simulink model "NFBLB_OSC_NON_LIN"  (R2021a)
settings: Solver=VariableStepAuto  StartTime=0.0  StopTime=85  RelTol=1e-3
model workspace (MATLAB code in the model file):
  | Kab=40;
  | Kia=0.5;
  | Kbc=20;
  | Fb=2;
  | kfb=1;
  | Kca=8;
  | Fc=0.5;
  | In=0.3;
  | x_star=[0.0069;0.5363;0.1000];
settings Model: Creator=priya  LastModifiedBy=Priyan_PC
settings SolverCC: AlgebraicLoopSolver=TrustRegion
settings DebuggingCC: SFMachineParentedDataDiag=warning

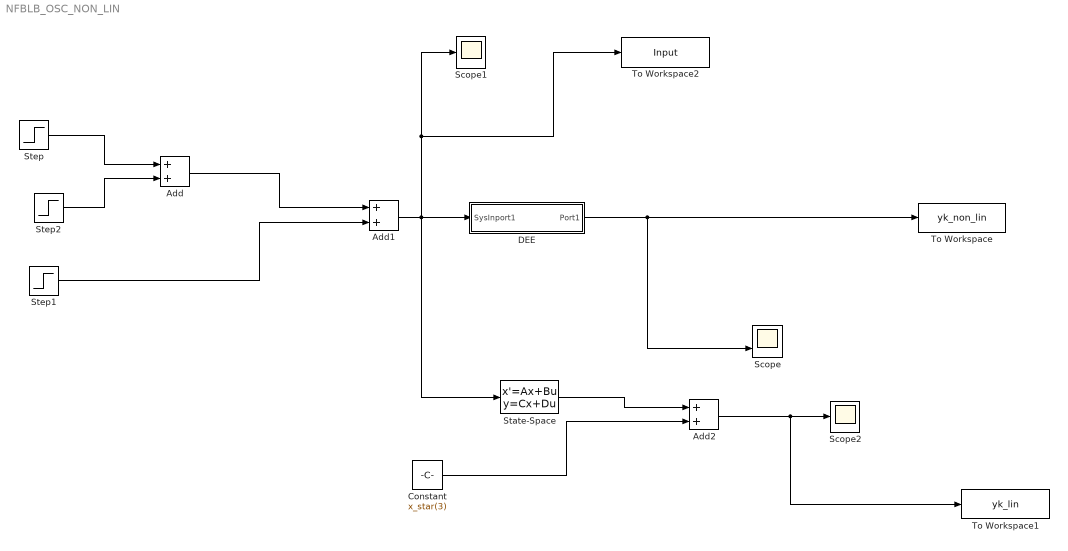
== system NFBLB_OSC_NON_LIN ==
  Add : Sum
  Add1 : Sum
  Add2 : Sum
  Constant : Constant  Value=x_star(3)
  DEE : Subsystem  mask(Differential Equation Editor (DEE)){}
      settings: OpenFcn=diffeqed
      mask Display: disp('Differential Equation\n Editor')
  Scope : Scope  NumInputPorts=2
  Scope1 : Scope
  Scope2 : Scope
  State-Space : StateSpace  A=[-21.4500 -0.2778 0;0 0 20;7.2 0 -0.5556];  B=[0.4965;0;0]  C=[0 0 1]  D=0  InitialCondition=0
  Step : Step  Time=0  Before=0.3  After=0.5  SampleTime=0
  Step1 : Step  Time=50  After=0.2  SampleTime=0
  Step2 : Step  Time=25  After=0.2  SampleTime=0
  To Workspace : ToWorkspace  VariableName=yk_non_lin  SampleTime=-1
  To Workspace1 : ToWorkspace  VariableName=yk_lin  SampleTime=-1
  To Workspace2 : ToWorkspace  VariableName=Input  SampleTime=-1
  wires:
  Add/1 -> Add1/1
  Add1/1 -> To Workspace2/1, Scope1/1, State-Space/1, DEE/1(SysInport1)
  Step1/1 -> Add1/2
  DEE/1(Port1) -> Scope/2, To Workspace/1
  Step/1 -> Add/1
  Step2/1 -> Add/2
  Constant/1 -> Add2/2
  State-Space/1 -> Add2/1
  Add2/1 -> To Workspace1/1, Scope2/1

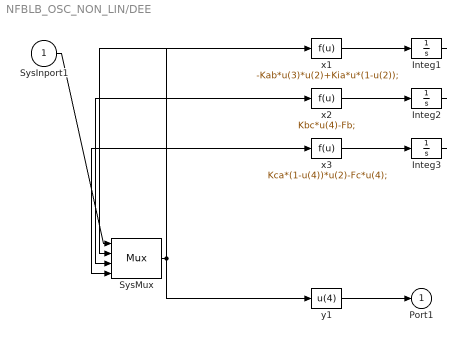
== system NFBLB_OSC_NON_LIN/DEE ==
  SysInport1 : Inport
  Integ1 : Integrator  InitialCondition=x_star(1)
  Integ2 : Integrator  InitialCondition=x_star(2)
  Integ3 : Integrator  InitialCondition=x_star(3)
  SysMux : Mux
  x1 : Fcn  Expr=-Kab*u(3)*u(2)+Kia*u*(1-u(2));
  x2 : Fcn  Expr=Kbc*u(4)-Fb;
  x3 : Fcn  Expr=Kca*(1-u(4))*u(2)-Fc*u(4);
  y1 : Fcn  Expr=u(4)
  Port1 : Outport
  wires:
  SysInport1/1 -> SysMux/1
  SysMux/1 -> x1/1, x2/1, x3/1, y1/1
  x1/1 -> Integ1/1
  Integ1/1 -> SysMux/2
  x2/1 -> Integ2/1
  Integ2/1 -> SysMux/3
  x3/1 -> Integ3/1
  Integ3/1 -> SysMux/4
  y1/1 -> Port1/1
